simulink model "Flexible_joints_manip_simulink_original_system_try"  (R2018b)
settings: Solver=FixedStepAuto  StartTime=0.0  StopTime=3  FixedStep=0.000001  RelTol=1e-3
settings Model: Creator=ahmed  LastModifiedBy=ahmed

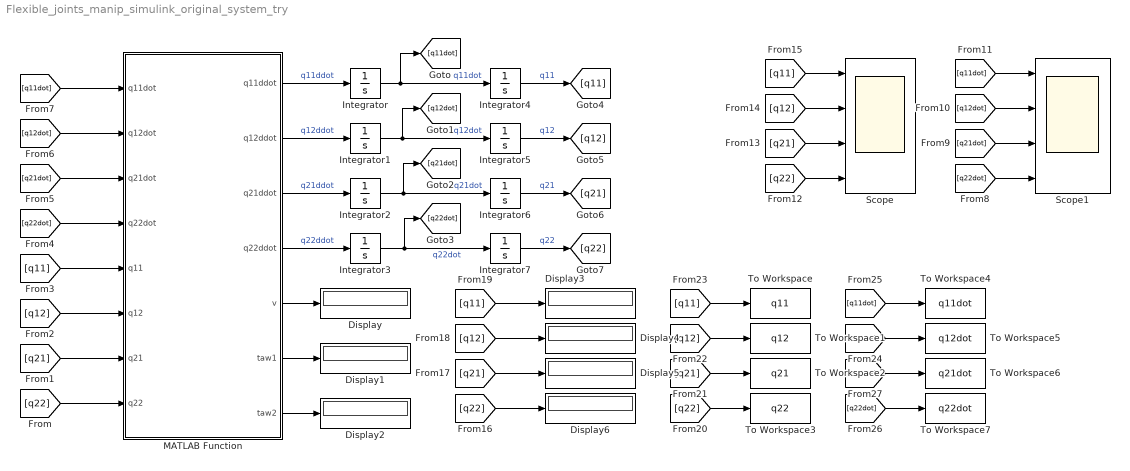
== system Flexible_joints_manip_simulink_original_system_try ==
  Display{,1..6} (7 alike) : Display
      settings: Decimation=4
  Integrator{,1..4,6} (6 alike) : Integrator
  Integrator5 : Integrator  InitialCondition=pi/4
  Integrator7 : Integrator  InitialCondition=pi/8
  MATLAB Function : MATLAB Function  TreatAsAtomicUnit=on
  Scope : Scope  NumInputPorts=4
  Scope1 : Scope  NumInputPorts=4
  To Workspace : ToWorkspace  VariableName=q11  SaveFormat=Timeseries  SampleTime=-1
  To Workspace1 : ToWorkspace  VariableName=q12  SaveFormat=Timeseries  SampleTime=-1
  To Workspace2 : ToWorkspace  VariableName=q21  SaveFormat=Timeseries  SampleTime=-1
  To Workspace3 : ToWorkspace  VariableName=q22  SaveFormat=Timeseries  SampleTime=-1
  To Workspace4 : ToWorkspace  VariableName=q11dot  SaveFormat=Timeseries  SampleTime=-1
  To Workspace5 : ToWorkspace  VariableName=q12dot  SaveFormat=Timeseries  SampleTime=-1
  To Workspace6 : ToWorkspace  VariableName=q21dot  SaveFormat=Timeseries  SampleTime=-1
  To Workspace7 : ToWorkspace  VariableName=q22dot  SaveFormat=Timeseries  SampleTime=-1
  wires:
  MATLAB Function/1(q11ddot) -> Integrator/1  "q11ddot"
  MATLAB Function/4(q22ddot) -> Integrator3/1  "q22ddot"
  MATLAB Function/3(q21ddot) -> Integrator2/1  "q21ddot"
  MATLAB Function/2(q12ddot) -> Integrator1/1  "q12ddot"
  Integrator/1 -> [q11dot], Integrator4/1  "q11dot"
  Integrator1/1 -> [q12dot], Integrator5/1  "q12dot"
  Integrator2/1 -> [q21dot], Integrator6/1  "q21dot"
  Integrator3/1 -> [q22dot], Integrator7/1  "q22dot"
  [q22] -> MATLAB Function/8(q22)
  [q21] -> MATLAB Function/7(q21)
  [q12] -> MATLAB Function/6(q12)
  [q11] -> MATLAB Function/5(q11)
  [q11dot] -> MATLAB Function/1(q11dot)
  [q12dot] -> MATLAB Function/2(q12dot)
  [q21dot] -> MATLAB Function/3(q21dot)
  [q22dot] -> MATLAB Function/4(q22dot)
  [q11dot] -> Scope1/1
  [q12dot] -> Scope1/2
  [q21dot] -> Scope1/3
  [q22dot] -> Scope1/4
  [q11] -> Scope/1
  [q12] -> Scope/2
  [q21] -> Scope/3
  [q22] -> Scope/4
  MATLAB Function/5(v) -> Display/1
  MATLAB Function/6(taw1) -> Display1/1
  MATLAB Function/7(taw2) -> Display2/1
  [q11] -> Display3/1
  [q12] -> Display4/1
  [q21] -> Display5/1
  [q22] -> Display6/1
  [q11] -> To Workspace/1
  [q12] -> To Workspace1/1
  [q21] -> To Workspace2/1
  [q22] -> To Workspace3/1
  [q11dot] -> To Workspace4/1
  [q12dot] -> To Workspace5/1
  [q21dot] -> To Workspace6/1
  [q22dot] -> To Workspace7/1
  Integrator4/1 -> [q11]  "q11"
  Integrator5/1 -> [q12]  "q12"
  Integrator6/1 -> [q21]  "q21"
  Integrator7/1 -> [q22]  "q22"

== matlab function Flexible_joints_manip_simulink_original_system_try/MATLAB Function ==
  data: q11ddot output; q12ddot output; q21ddot output; q22ddot output; q11dot input; q12dot input; q21dot input; q22dot input; q11 input; q12 input; q21 input; q22 input; v output; taw1 output; taw2 output
function [q11ddot,q12ddot,q21ddot,q22ddot,v,taw1,taw2]= fcn(q11dot,q12dot,q21dot,q22dot,q11,q12,q21,q22)

p1 = 1.5; p2 = 0.5; p3 = 2; p4 = 0.2; p5 = 1; p6 = 1; p7 = 50;
k1 = 100; k2 = 200;

M1 = [p1+p2*cos(q12)^2 0; 0 p3];
M2 = [0 p4; 0 0];
M3 = [p5 0; 0 p6];
M = [M1 M2; M2' M3];

x1 = q11; x2 = q11dot; x3 = q12; x4 = q12dot;
x5 = q22; x6 = q22dot; x7 = q21; x8 = q21dot;

% x2 = e2-x1;
% x3 = e3-2*e2;
% x4 = e4-3*e3+e2+2*x1;

e2 = x2 + x1;
e3 = x3 + 2*e2;
e4 = x4 + 3*e3 - e2 - 2*x1;
e5 = (k2/p3)*x5 + 4*e4 - (3+(k2/p3))*e3 - (4-2*(k2/p3))*e2 + 3*x1 ...
     - (p7/p3)*cos(e3-2*e2) ...
     - (p2/(2*p3))*(e2-x1)^2*sin(2*(e3-2*e2));

e6 = (k2/p3)*x6 + 5*e5 - (6+(k2/p3))*e4 - (5-3*(k2/p3))*e3 ...
     + (10-(k2/p3))*e2 + (1-2*(k2/p3))*x1 ...
     + (p7/p3)*(e4-3*e3+e2+2*x1)*sin(e3-2*e2) ...
     - (p2/p3)*(e2-x1)*(e3-2*e2)*sin(2*(e3-2*e2)) ...
     - (p2/p3)*(e2-x1)^2*(e4-3*e3+e2+2*x1)*cos(2*(e3-2*e2));

e7 = (k1*k2/(p3*p4))*x7 + 6*e6 - (10+(k2/p3))*e5 - (4-4*(k2/p3))*e4 ...
     + (21-3*(k2/p3)-(p1*k2/(p3*p4)))*e3 ...
     - (4+4*(k2/p3)-2*(p1*k2/(p3*p4)))*e2 ...
     - (11-3*(k2/p3)+(k1*k2/(p3*p4)))*x1 ...
     + (k2*p2/(p3*p4))*(e2-x1)*(e4-3*e3+e2+2*x1)*sin(2*(e3-2*e2)) ...
     - (k2*p2/(p3*p4))*(e3-2*e2)*cos(e3-2*e2)^2 ...
     + (p7/p3)*(e4-3*e3+e2+2*x1)^2*cos(e3-2*e2) ...
     + (p7/p3)*(e5-4*e4+3*e3+4*e2-3*x1)*sin(e3-2*e2) ...
     - (2*p2/p3)*(e2-x1)*(e3-2*e2)*(e4-3*e3+e2+2*x1)*cos(2*(e3-2*e2)) ...
     - (p2/p3)*(e2-x1)*(e4-3*e3+e2+2*x1)*sin(2*(e3-2*e2)) ...
     - (p2/p3)*(e3-2*e2)^2*sin(2*(e3-2*e2)) ...
     + (2*p2/p3)*(e2-x1)^2*(e4-3*e3+e2+2*x1)^2*sin(2*(e3-2*e2)) ...
     - (p2/p3)*(e2-x1)^2*(e5-4*e4+3*e3+4*e2-3*x1)*cos(2*(e3-2*e2)) ...
     - (2*p2/p3)*(e2-x1)*(e3-2*e2)*(e4-3*e3+e2+2*x1)*cos(2*(e3-2*e2));

% (e2-x1)
% (e3-2*e2)
% (e4-3*e3+e2+2*x1)
% (e5-4*e4+3*e3+4*e2-3*x1)
% (e6-5*e5+6*e4+5*e3-10*e2-x1)
% (e7-6*e6+10*e5+4*e4-21*e3+4*e2+11*x1)
% ((k2*p2-p4*p2)/(p3*p4))
% (k2*p2/(p3*p4))
% (p7/p3)
% (p2/p3)

phidot = -(k2*p2/(p3*p4))*(e4-3*e3+e2+2*x1)*cos(e3-2*e2)^2 ...
     - (p7/p3)*(e4-3*e3+e2+2*x1)^3*sin(e3-2*e2) ...
     + (p7/p3)*(e6-5*e5+6*e4+5*e3-10*e2-x1)*sin(e3-2*e2) ...
     + (3*p7/p3)*(e4-3*e3+e2+2*x1)*(e5-4*e4+3*e3+4*e2-3*x1)*cos(e3-2*e2) ...
     + ((2*k2*p2-3*p4*p2)/(p3*p4))*(e3-2*e2)*(e4-3*e3+e2+2*x1)*sin(2*(e3-2*e2)) ...
     + ((k2*p2-p4*p2)/(p3*p4))*(e2-x1)*(e5-4*e4+3*e3+4*e2-3*x1)*sin(2*(e3-2*e2)) ...
     + (12*p2/p3)*(e2-x1)*(e3-2*e2)*(e4-3*e3+e2+2*x1)^2*sin(2*(e3-2*e2)) ...
     + (6*p2/p3)*(e2-x1)^2*(e4-3*e3+e2+2*x1)*(e5-4*e4+3*e3+4*e2-3*x1)*sin(2*(e3-2*e2)) ...
     + (4*p2/p3)*(e2-x1)^2*(e4-3*e3+e2+2*x1)^3*cos(2*(e3-2*e2)) ...
     - (p2/p3)*(e2-x1)^2*(e6-5*e5+6*e4+5*e3-10*e2-x1)*cos(2*(e3-2*e2)) ...
     + ((2*k2*p2-6*p4*p2)/(p3*p4))*(e2-x1)*(e4-3*e3+e2+2*x1)^2*cos(2*(e3-2*e2)) ...
     - (6*p2/p3)*(e2-x1)*(e3-2*e2)*(e5-4*e4+3*e3+4*e2-3*x1)*cos(2*(e3-2*e2)) ...
     - (6*p2/p3)*(e3-2*e2)^2*(e4-3*e3+e2+2*x1)*cos(2*(e3-2*e2));

e8 = (k1*k2/(p3*p4))*x8 + 7*e7 - (15+(k2/p3))*e6 + 5*(k2/p3)*e5 ...
     + (35-6*(k2/p3)-(p1*k2/(p3*p4)))*e4 ...
     - (21+5*(k2/p3)-3*(p1*k2/(p3*p4)))*e3 ...
     - (28-10*(k2/p3)+(p1*k2/(p3*p4))+(k1*k2/(p3*p4)))*e2 ...
     + (15+(k2/p3)-2*(p1*k2/(p3*p4))+(k1*k2/(p3*p4)))*x1 ...
     + phidot;

phiddot = -(k2*p2/(p3*p4))*(e5-4*e4+3*e3+4*e2-3*x1)*cos(e3-2*e2)^2 ...
     - (p7/p3)*(e4-3*e3+e2+2*x1)^4*cos(e3-2*e2) ...
     + (3*p7/p3)*(e5-4*e4+3*e3+4*e2-3*x1)^2*cos(e3-2*e2) ...
     + (4*p7/p3)*(e4-3*e3+e2+2*x1)*(e6-5*e5+6*e4+5*e3-10*e2-x1)*cos(e3-2*e2) ...
     - (6*p7/p3)*(e4-3*e3+e2+2*x1)^2*(e5-4*e4+3*e3+4*e2-3*x1)*sin(e3-2*e2) ...
     + (p7/p3)*(e7-6*e6+10*e5+4*e4-21*e3+4*e2+11*x1)*sin(e3-2*e2) ...
     + ((3*k2*p2-3*p4*p2)/(p3*p4))*(e4-3*e3+e2+2*x1)^2*sin(2*(e3-2*e2)) ...
     + ((3*k2*p2-4*p4*p2)/(p3*p4))*(e3-2*e2)*(e5-4*e4+3*e3+4*e2-3*x1)*sin(2*(e3-2*e2)) ...
     + ((6*k2*p2-24*p4*p2)/(p3*p4))*(e3-2*e2)*(e4-3*e3+e2+2*x1)^2*cos(2*(e3-2*e2)) ...
     + ((k2*p2-p4*p2)/(p3*p4))*(e2-x1)*(e6-5*e5+6*e4+5*e3-10*e2-x1)*sin(2*(e3-2*e2)) ...
     + (48*p2/p3)*(e2-x1)*(e3-2*e2)*(e4-3*e3+e2+2*x1)*(e5-4*e4+3*e3+4*e2-3*x1)*sin(2*(e3-2*e2)) ...
     - ((4*k2*p2-24*p4*p2)/(p3*p4))*(e2-x1)*(e4-3*e3+e2+2*x1)^3*sin(2*(e3-2*e2)) ...
     + (24*p2/p3)*(e3-2*e2)^2*(e4-3*e3+e2+2*x1)^2*sin(2*(e3-2*e2)) ...
     + (8*p2/p3)*(e2-x1)^2*(e4-3*e3+e2+2*x1)*(e6-5*e5+6*e4+5*e3-10*e2-x1)*sin(2*(e3-2*e2)) ...
     + (6*p2/p3)*(e2-x1)^2*(e5-4*e4+3*e3+4*e2-3*x1)^2*sin(2*(e3-2*e2)) ...
     - (8*p2/p3)*(e2-x1)^2*(e4-3*e3+e2+2*x1)^4*sin(2*(e3-2*e2)) ...
     + ((6*k2*p2-20*p4*p2)/(p3*p4))*(e2-x1)*(e4-3*e3+e2+2*x1)*(e5-4*e4+3*e3+4*e2-3*x1)*cos(2*(e3-2*e2)) ...
     + (32*p2/p3)*(e2-x1)*(e3-2*e2)*(e4-3*e3+e2+2*x1)^3*cos(2*(e3-2*e2)) ...
     + (24*p2/p3)*(e2-x1)^2*(e4-3*e3+e2+2*x1)^2*(e5-4*e4+3*e3+4*e2-3*x1)*cos(2*(e3-2*e2)) ...
     - (p2/p3)*(e2-x1)^2*(e7-6*e6+10*e5+4*e4-21*e3+4*e2+11*x1)*cos(2*(e3-2*e2)) ...
     - (8*p2/p3)*(e2-x1)*(e3-2*e2)*(e6-5*e5+6*e4+5*e3-10*e2-x1)*cos(2*(e3-2*e2)) ...
     - (12*p2/p3)*(e3-2*e2)^2*(e5-4*e4+3*e3+4*e2-3*x1)*cos(2*(e3-2*e2));
  
v = (p3*p4/(k1*k2))*(-8*e8 + (21+(k2/p3))*e7 - (8+6*(k2/p3))*e6 ...
    - (50-10*(k2/p3)-(p1*k2/(p3*p4)))*e5 ...
    + (56+4*(k2/p3)-4*(p1*k2/(p3*p4)))*e4 ...
    + (42-21*(k2/p3)+3*(p1*k2/(p3*p4))+(k1*k2/(p3*p4)))*e3 ...
    - (64-4*(k2/p3)-4*(p1*k2/(p3*p4))+2*(k1*k2/(p3*p4)))*e2 ...
    - (13-11*(k2/p3)+3*(p1*k2/(p3*p4)))*x1 ...
    + phiddot);

taw1 = k1*(q21-q11)+p5*v;
taw2 = (-1/p4)*(p2*p6*q12*cos(q12)^2-p2*p6*q11dot*q12dot*sin(2*q12)...
       +k2*p4*q12+p1*p6*q12-k2*p4*q22+k1*p6*q11-k1*p6*q21-p4^2*q12);

taw = [0; 0; taw1; taw2];
C = [-p2*q11dot*q12dot*sin(2*q12); 0.5*p2*q11dot^2*sin(2*q12); 0; 0];
K = [k1*(q11-q21); k2*(q12-q22); k1*(q21-q11); k2*(q22-q12)];
G = [0; p7*cos(q12); 0; 0];
q = M^-1*(taw-C-K-G);

q11ddot=q(1);
q12ddot=q(2);
q21ddot=q(3);
q22ddot=q(4);
